simulink model "cassie"  (R2017b)
settings: Solver=FixedStepAuto  StartTime=0.0  StopTime=inf  RelTol=1e-3
InitFcn:
  | PreFunctions.PreParams
undefined symbols (not defined in the file or in its folder): UserParams
libraries: xpcethercatlib x47, ComponentLibrary x10, slrtlib x5, xpcutilitieslib x2, xpcrtudplib x2, dsparch4 x2
(part 1 of 2)
settings Model: xpc_rtwmakecfg_data=_xpcethercatlib_  SimulationMode=external  Creator=hanli  LastModifiedBy=Robot
settings SolverCC: ConcurrentTasks=on  AutoInsertRateTranBlk=on
settings DataIOCC: SaveFormat=StructureWithTime
settings OptimizationCC: BlockReduction=off  SimCompilerOptimization=on  AccelVerboseBuild=on
settings DebuggingCC: InheritedTsInSrcMsg=none
settings HardwareCC: ProdBitPerPointer=32  ProdBitPerSizeT=32  ProdBitPerPtrDiffT=32  ProdLargestAtomicFloat=None  ProdWordSize=32  ProdLongLongMode=on  ProdHWDeviceType=Generic->32-bit x86 compatible
settings RTWCC: SystemTargetFile=slrt.tlc  TemplateMakefile=slrt_default_tmf  Description=Simulink Real-Time  CustomSource=Jp_toe_joint_right_src.c  CodeExecutionProfiling=on  RTWCompilerOptimization=on
settings SimulinkRealTimeCC: SupportVariableSizeSignals=on  RL32LogTETModifier=off  xPCConcurrentTasks=on

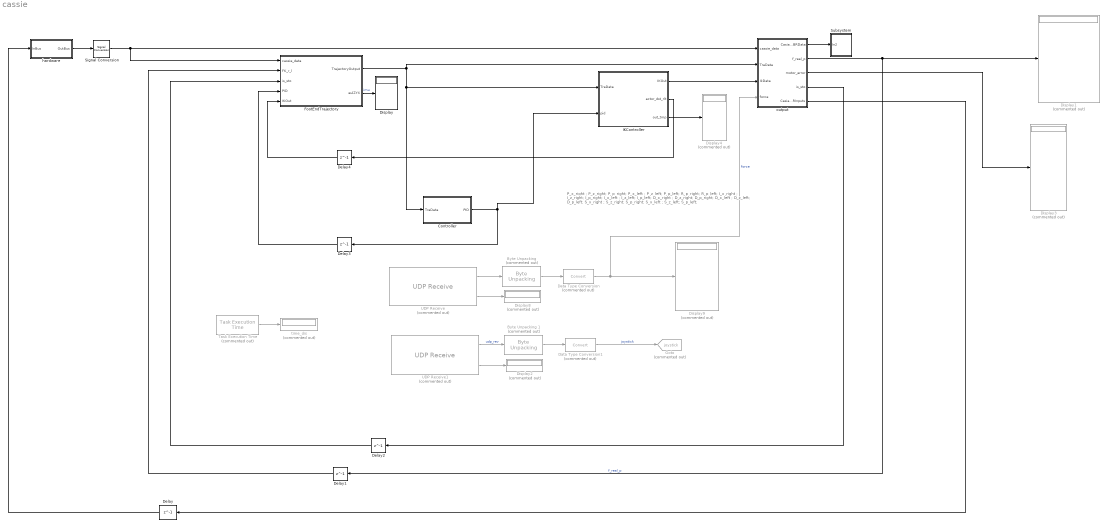
== system cassie ==
  note: P_x_right ; P_z_right; P_p_right; P_x_left ; P_z_left; P_p_left; R_p_right; R_p_left;
      |
      | I_x_right ;   I_z_right;  I_p_right;  I_x_left ; I_z_left;  I_p_left;
      |
      | D_x_right ; D_z_right; D_p_right; D_x_left ; D_z_left; D_p_left;
      |
      | S_x_right ; S_z_right; S_p_right; S_x_left ; S_z_left; S_p_left;
  "Byte Unpacking " : xpcutilitieslib/Byte Unpacking   Commented=on  MaskUnpackedDataTypes={'single'}  MaskUnpackedDataSizes={[6]}  MaskAlignment=1
      settings: SourceProductName=Simulink Real-Time  SourceProductBaseCode=XP
  Byte Unpacking 1 : xpcutilitieslib/Byte Unpacking   Commented=on  MaskUnpackedDataTypes={'int8'}  MaskUnpackedDataSizes={[11]}  MaskAlignment=1
      settings: SourceProductName=Simulink Real-Time  SourceProductBaseCode=XP
  Controller : Subsystem
  Data Type Conversion : DataTypeConversion  Commented=on
  Data Type Conversion1 : DataTypeConversion  Commented=on
  Delay{,1..4} (5 alike) : Delay  DelayLength=1  InitialCondition=0
  Display : Display
  Display{1..4,8..9} (6 alike) : Display  Commented=on
  FootEndTrajectory : Subsystem
  Goto : Goto  Commented=on  GotoTag=joystick  TagVisibility=global
  IKController : Subsystem
  Signal Conversion : SignalConversion  ConversionOutput=Nonvirtual bus  OutDataTypeStr=Bus: CassieOutBus  OverrideOpt=off
  Subsystem : Subsystem
  "Task Execution Time " : slrtlib/Target Management/Execution Parameters/Task Execution Time   Commented=on  ts=1/2000
      settings: SourceProductName=Simulink Real-Time  SourceProductBaseCode=XP
  UDP Receive : xpcrtudplib/UDP Receive  Commented=on  ipAddressVal=Use host-target connection  localPort=10001  rcvWidth=24  rcvFmAny=on  fmAddress=0.0.0.0  maxUDPQueue=8  sampleTime=0.001
      settings: SourceProductName=Simulink Real-Time
  UDP Receive1 : xpcrtudplib/UDP Receive  Commented=on  ipAddressVal=Use host-target connection  localPort=10001  rcvWidth=11  rcvFmAny=on  fmAddress=0.0.0.0  maxUDPQueue=8  sampleTime=0.005
      settings: SourceProductName=Simulink Real-Time
  hardware : Subsystem  InitFcn=PreFunctions.BusInfos
  output : Subsystem
  time_dis : Display  Commented=on
  wires:
  hardware/1(OutBus) -> Signal Conversion/1
  Delay/1 -> hardware/1(InBus)
  Signal Conversion/1 -> FootEndTrajectory/1(cassie_data), output/1(cassie_data)
  output/3(motor_error) -> Display3/1
  "Task Execution Time "/1 -> time_dis/1
  FootEndTrajectory/1(TrajectoryOutput) -> output/2(TraData), Controller/1(TraData), IKController/1(TraData)
  Delay1/1 -> FootEndTrajectory/2(FK_r_l)
  Delay2/1 -> FootEndTrajectory/3(is_sto)
  FootEndTrajectory/2(eulZYX) -> Display/1  "imu"
  Controller/1(PID) -> IKController/2(pid), Delay3/1
  output/2(f_real_p) -> Delay1/1, Display1/1  "f_real_p"
  IKController/1(IKOut) -> output/3(IkData)
  output/1(CasiaBBRData) -> Subsystem/1(In2)
  output/5(CasiaBBRInputs) -> Delay/1
  output/4(is_sto) -> Delay2/1
  UDP Receive/1 -> "Byte Unpacking "/1
  "Byte Unpacking "/1 -> Data Type Conversion/1
  UDP Receive/2 -> Display8/1
  Data Type Conversion/1 -> output/4(force), Display9/1  "force"
  IKController/3(out_tmp) -> Display4/1
  Delay3/1 -> FootEndTrajectory/4(PID)
  UDP Receive1/1 -> Byte Unpacking 1/1  "udp_rev"
  UDP Receive1/2 -> Display2/1
  Byte Unpacking 1/1 -> Data Type Conversion1/1
  Data Type Conversion1/1 -> Goto/1  "joystick"
  Delay4/1 -> FootEndTrajectory/5(IKOut)
  IKController/2(actor_dst_rlt) -> Delay4/1

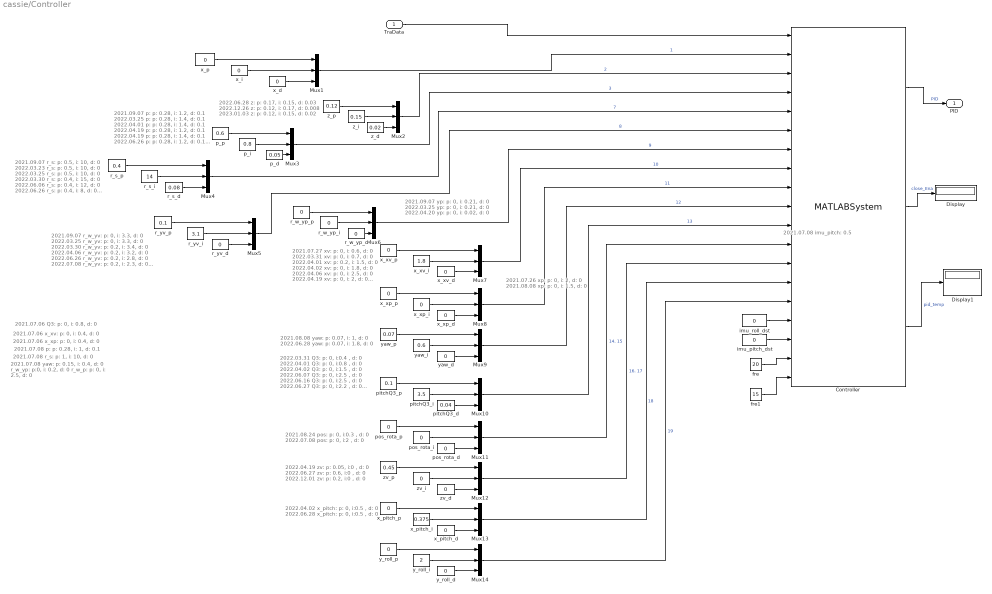
== system cassie/Controller ==
  note: 2021.07.06 x_xp: p: 0, i: 0.4, d: 0
  note: 2021.07.06 x_xv: p: 0, i: 0.4, d: 0
  note: 2021.07.06 Q3: p: 0, i: 0.8, d: 0
  note: 2021.07.08 imu_pitch: 0.5
  note: 2021.07.08 p: p: 0.28, i: 1, d: 0.1
  note: 2021.07.08 r_s: p: 1, i: 10, d: 0
  note: 2021.07.08    yaw: p: 0.15, i: 0.4, d: 0
      |                    r_w_yp: p:0, i: 0.2, d: 0
      |    			r_w_p: p: 0, i: 2.5, d: 0
  note: 2021.07.26     xp: p: 0, i: 2, d: 0
      | 2021.08.08     xp: p: 0, i: 1.5, d: 0
  note: 2021.07.27     xv: p: 0, i: 0.6, d: 0
      | 2022.03.31     xv: p: 0, i: 0.7, d: 0
      | 2022.04.01     xv: p: 0.2, i: 1.5, d: 0
      | 2022.04.02     xv: p: 0, i: 1.8, d: 0
      | 2022.04.06     xv: p: 0, i: 2.5, d: 0
      | 2022.04.19     xv: p: 0, i: 2, d: 0
      | 2022.06.08     xv: p: 0, i: 2, d: 0
      | 2022.06.16     xv: p: 0, i: 2.5, d: 0
      | 2022.06.26     xv: p: 0, i: 2.5, d: 0
      | 2022.07.08     xv: p: 0, i: 1.7, d: 0
  note: 2021.08.08     yaw: p: 0.07, i: 1, d: 0
      | 2022.06.28     yaw: p: 0.07, i: 1.8, d: 0
  note: 2021.09.07     yp: p: 0, i: 0.21, d: 0
      | 2022.03.25     yp: p: 0, i: 0.21, d: 0
      | 2022.04.20     yp: p: 0, i: 0.02, d: 0
  note: 2021.09.07    r_s: p: 0.5, i: 10, d: 0
      | 2022.03.23    r_s: p: 0.5, i: 10, d: 0
      | 2022.03.25    r_s: p: 0.5, i: 10, d: 0
      | 2022.03.30    r_s: p: 0.4, i: 15, d: 0
      | 2022.06.06    r_s: p: 0.4, i: 12, d: 0
      | 2022.06.26    r_s: p: 0.4, i: 8, d: 0
      | 2022.06.28    r_s: p: 0.4, i: 12, d: 0
      | 2022.11.24    r_s: p: 0.4, i: 12, d: 0
      | 2022.12.08    r_s: p: 0.7, i: 16, d: 0.12
      | 2022.12.22    r_s: p: 0.4, i: 16, d: 0.12
      | 2022.12.26    r_s: p: 0.4, i: 14, d: 0.06
  note: 2021.08.24    pos: p: 0, i:0.3 , d: 0
      | 2022.07.08    pos: p: 0, i:2 , d: 0
  note: 2021.09.07     p: p: 0.28, i: 1.2, d: 0.1
      | 2022.03.25     p: p: 0.28, i: 1.4, d: 0.1
      | 2022.04.01     p: p: 0.28, i: 1.4, d: 0.1
      | 2022.04.19     p: p: 0.28, i: 1.2, d: 0.1
      | 2022.04.19     p: p: 0.28, i: 1.4, d: 0.1
      | 2022.06.26     p: p: 0.28, i: 1.2, d: 0.1
      | 2022.06.28     p: p: 0.25, i: 1.4, d: 0.1
  note: 2021.09.07    r_w_yv: p: 0, i: 3.3, d: 0
      | 2022.03.25    r_w_yv: p: 0, i: 3.3, d: 0
      | 2022.03.30    r_w_yv: p: 0.2, i: 3.4, d: 0
      | 2022.04.06    r_w_yv: p: 0.2, i: 3.2, d: 0
      | 2022.06.26    r_w_yv: p: 0.2, i: 2.8, d: 0
      | 2022.07.08    r_w_yv: p: 0.2, i: 2.3, d: 0
      | 2022.08.08    r_w_yv: p: 0.2, i: 2.2, d: 0
      | 2022.12.26    r_w_yv: p: 0, i: 4.2, d: 0
  note: 2022.03.31     Q3: p: 0, i:0.4 , d: 0
      | 2022.04.01     Q3: p: 0, i:0.8 , d: 0
      | 2022.04.02     Q3: p: 0, i:1.5 , d: 0
      | 2022.06.07     Q3: p: 0, i:2.5 , d: 0
      | 2022.06.16     Q3: p: 0, i:2.5 , d: 0
      | 2022.06.27     Q3: p: 0, i:2.2 , d: 0
      | 2022.07.08     Q3: p: 0, i:1.8 , d: 0
      | 2022.12.02     Q3: p: 0, i:2.7 , d: 0
      | 2022.12.07     Q3: p: 0, i:4 , d: 0
      | 2022.12.26     Q3: p: 0.1, i:4 , d: 0.035
  note: 2022.04.02    x_pitch: p: 0, i:0.5 , d: 0
      | 2022.06.28    x_pitch: p: 0, i:0.5 , d: 0
  note: 2022.04.19    zv: p: 0.05, i:0 , d: 0
      | 2022.06.27    zv: p: 0.6, i:0 , d: 0
      | 2022.12.01    zv: p: 0.2, i:0 , d: 0
  note: 2022.06.28     z: p: 0.17, i: 0.15, d: 0.03
      | 2022.12.26     z: p: 0.12, i: 0.17, d: 0.008
      | 2023.01.03     z: p: 0.12, i: 0.15, d: 0.02
  TraData : Inport
  Controller : MATLABSystem  System=Controller  SimulateUsing=Code generation
      mask Type: Controller
      mask Display:
      | disp('Controller');
      | port_label('input',1,'TraData');
      | port_label('input',2,'x_pid');
      | port_label('input',3,'z_pid');
      | port_label('input',4,'p_pid');
      | port_label('input',5,'r_st_pid');
      | port_label('input',6,'yv_pid');
      | port_label('input',7,'yp_pid');
      | port_label('input',8,'xv_pid');
      | port_label('input',9,'xp_pid');
      | port_label('input',10,'yaw_pid');
      | port_label('input',11,'q3_pid');
      | port_label('input',12,'pos_rota_pid');
      | port_label('input',13,'zv_pid');
      | port_label('input',14,'x_pitch_pid');
      | port_label('input',15,'y_roll_pid');
      | port_label('input',16,'imu_roll_dst');
      | port_label('input',17,'imu_pitch_dst');
      | port_label('input',18,'fre_roll');
      | port_label('input',19,'fre_pitch');
      | port_label('output',1,'pid_out');
      | port_label('output',2,'closedloop_Ena');
      | port_label('output',3,'pid_tmp');
  Display : Display
  Display1 : Display
  Mux{1..14} (14 alike) : Mux  Inputs=3
  fre : Constant  Value=20
  fre1 : Constant  Value=15
  imu_pitch_dst : Constant  Value=0
  imu_roll_dst : Constant  Value=0
  p_d : Constant  Value=0.05
  p_i : Constant  Value=0.8
  p_p : Constant  Value=0.6
  pitchQ3_d : Constant  Value=0.04
  pitchQ3_i : Constant  Value=3.5
  pitchQ3_p : Constant  Value=0.1
  pos_rota_d : Constant  Value=0
  pos_rota_i : Constant  Value=0
  pos_rota_p : Constant  Value=0
  r_s_d : Constant  Value=0.08
  r_s_i : Constant  Value=14
  r_s_p : Constant  Value=0.4
  r_w_yp_d : Constant  Value=0
  r_w_yp_i : Constant  Value=0
  r_w_yp_p : Constant  Value=0
  r_yv_d : Constant  Value=0
  r_yv_i : Constant  Value=3.1
  r_yv_p : Constant  Value=0.1
  x_d : Constant  Value=0
  x_i : Constant  Value=0
  x_p : Constant  Value=0
  x_pitch_d : Constant  Value=0
  x_pitch_i : Constant  Value=0.375
  x_pitch_p : Constant  Value=0
  x_xp_d : Constant  Value=0
  x_xp_i : Constant  Value=0
  x_xp_p : Constant  Value=0
  x_xv_d : Constant  Value=0
  x_xv_i : Constant  Value=1.8
  x_xv_p : Constant  Value=0
  y_roll_d : Constant  Value=0
  y_roll_i : Constant  Value=2
  y_roll_p : Constant  Value=0
  yaw_d : Constant  Value=0
  yaw_i : Constant  Value=0.6
  yaw_p : Constant  Value=0.07
  z_d : Constant  Value=0.02
  z_i : Constant  Value=0.15
  z_p : Constant  Value=0.12
  zv_d : Constant  Value=0
  zv_i : Constant  Value=0
  zv_p : Constant  Value=0.45
  PID : Outport
  wires:
  Mux2/1 -> Controller/3  "2"
  p_p/1 -> Mux3/1
  z_p/1 -> Mux2/1
  z_d/1 -> Mux2/3
  z_i/1 -> Mux2/2
  Mux1/1 -> Controller/2  "1"
  p_i/1 -> Mux3/2
  x_p/1 -> Mux1/1
  Controller/1 -> PID/1  "PID"
  x_d/1 -> Mux1/3
  p_d/1 -> Mux3/3
  Mux3/1 -> Controller/4  "3"
  x_i/1 -> Mux1/2
  TraData/1 -> Controller/1
  r_s_d/1 -> Mux4/3
  r_s_i/1 -> Mux4/2
  Mux4/1 -> Controller/5  "7"
  r_s_p/1 -> Mux4/1
  r_yv_p/1 -> Mux5/1
  r_yv_d/1 -> Mux5/3
  r_yv_i/1 -> Mux5/2
  Mux5/1 -> Controller/6  "8"
  Controller/2 -> Display/1  "close_Ena"
  Mux8/1 -> Controller/9  "11"
  x_xv_p/1 -> Mux7/1
  x_xp_i/1 -> Mux8/2
  x_xp_p/1 -> Mux8/1
  x_xp_d/1 -> Mux8/3
  Mux7/1 -> Controller/8  "10"
  r_w_yp_p/1 -> Mux6/1
  r_w_yp_i/1 -> Mux6/2
  Mux6/1 -> Controller/7  "9"
  x_xv_i/1 -> Mux7/2
  r_w_yp_d/1 -> Mux6/3
  x_xv_d/1 -> Mux7/3
  yaw_p/1 -> Mux9/1
  yaw_d/1 -> Mux9/3
  Mux9/1 -> Controller/10  "12"
  yaw_i/1 -> Mux9/2
  Mux10/1 -> Controller/11  "13"
  pitchQ3_d/1 -> Mux10/3
  pitchQ3_i/1 -> Mux10/2
  pitchQ3_p/1 -> Mux10/1
  pos_rota_d/1 -> Mux11/3
  pos_rota_i/1 -> Mux11/2
  pos_rota_p/1 -> Mux11/1
  Mux11/1 -> Controller/12  "14. 15"
  zv_d/1 -> Mux12/3
  Mux12/1 -> Controller/13  "16. 17"
  zv_p/1 -> Mux12/1
  zv_i/1 -> Mux12/2
  x_pitch_p/1 -> Mux13/1
  x_pitch_d/1 -> Mux13/3
  Mux13/1 -> Controller/14  "18"
  x_pitch_i/1 -> Mux13/2
  Controller/3 -> Display1/1  "pid_temp"
  imu_roll_dst/1 -> Controller/16
  imu_pitch_dst/1 -> Controller/17
  fre/1 -> Controller/18
  fre1/1 -> Controller/19
  y_roll_p/1 -> Mux14/1
  Mux14/1 -> Controller/15  "19"
  y_roll_d/1 -> Mux14/3
  y_roll_i/1 -> Mux14/2

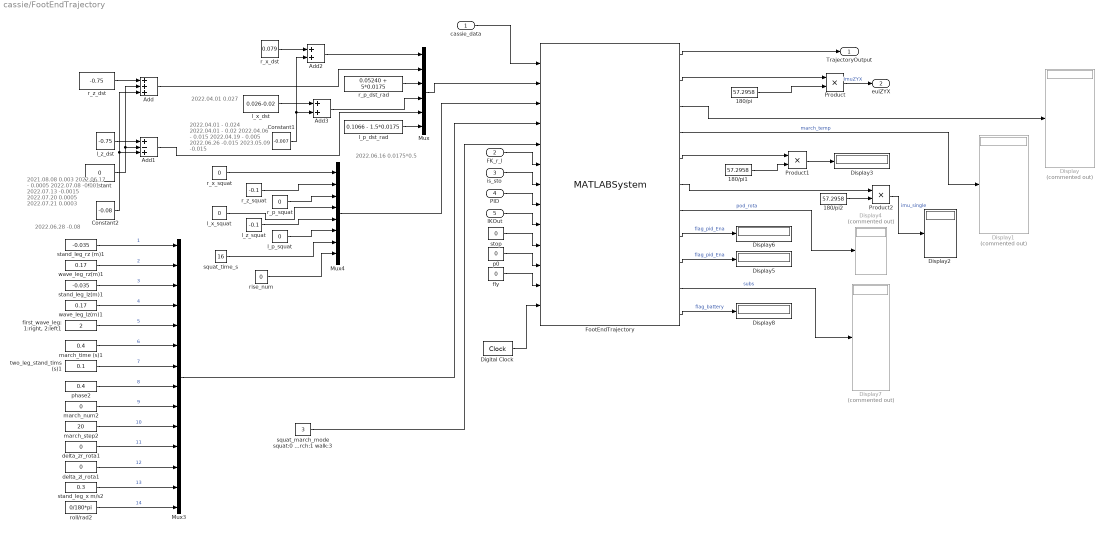
== system cassie/FootEndTrajectory ==
  note: 2021.08.08    0.003
      | 2022.06.17   - 0.0005
      | 2022.07.08   -0.001
      | 2022.07.13   -0.0015
      | 2022.07.20   0.0005
      | 2022.07.21   0.0003
  note: 2022.04.01   - 0.024
      | 2022.04.01   - 0.02
      | 2022.04.06   - 0.015
      | 2022.04.19   - 0.005
      | 2022.06.26    -0.015
      | 2023.05.09    -0.015
  note: 2022.04.01 0.027
  note: 2022.06.16 0.0175*0.5
  note: 2022.06.28 -0.08
  cassie_data : Inport
  FK_r_l : Inport  Port=2
  is_sto : Inport  Port=3
  PID : Inport  Port=4
  IKOut : Inport  Port=5
  180/pi : Constant  Value=57.2958
  180/pi1 : Constant  Value=57.2958
  180/pi2 : Constant  Value=57.2958
  Add : Sum  Inputs=+++
  Add1 : Sum  Inputs=+-+
  Add2 : Sum
  Add3 : Sum
  Constant : Constant  Value=0
  Constant1 : Constant  Value=-0.007
  Constant2 : Constant  Value=-0.08
  Digital Clock : DigitalClock  SampleTime=UserParams.SampleTime
  Display{,1,4,7} (4 alike) : Display  Commented=on
  Display{2..3,5..6,8} (5 alike) : Display
  FootEndTrajectory : MATLABSystem  System=FootEndTrajectory  SimulateUsing=Code generation
      mask Type: FootEndTrajectory
      mask Display:
      | disp('FootEndTrajectory');
      | port_label('input',1,'cassie_data');
      | port_label('input',2,'IK_tgt');
      | port_label('input',3,'squat');
      | port_label('input',4,'march');
      | port_label('input',5,'op_mode');
      | port_label('input',6,'FK_r_l');
      | port_label('input',7,'is_sto');
      | port_label('input',8,'pid_out');
      | port_label('input',9,'actor_dst_rlt');
      | port_label('input',10,'flag_stop');
      | port_label('input',11,'flag_p0');
      | port_label('input',12,'flag_fly');
      | port_label('input',13,'t');
      | port_label('output',1,'TrajectotyOutput');
      | port_label('output',2,'eulZYX');
      | port_label('output',3,'IK_dst');
      | port_label('output',4,'march_temp');
      | port_label('output',5,'yaw0');
      | port_label('output',6,'eulZYX_single');
      | port_label('output',7,'pos_rota');
      | port_label('output',8,'t_pid_Ena');
      | port_label('output',9,'flag_pid_Ena');
      | port_label('output',10,'controller');
      | port_label('output',11,'flag_battery');
  Mux : Mux  Inputs=6
  Mux3 : Mux  Inputs=14
  Mux4 : Mux  Inputs=8
  Product : Product
  Product1 : Product
  Product2 : Product
  delta_zl_rota1 : Constant  Value=0
  delta_zr_rota1 : Constant  Value=0
  "first_wave_leg: 1:right, 2:left1" : Constant  Value=2
  fly : Constant  Value=0
  l_p_dst_rad : Constant  Value=0.1066 - 1.5*0.0175
  l_p_squat : Constant  Value=0
  l_x_dst : Constant  Value=0.026-0.02
  l_x_squat : Constant  Value=0
  l_z_dst : Constant  Value=-0.75
  l_z_squat : Constant  Value=-0.1
  march_num2 : Constant  Value=0
  march_step2 : Constant  Value=20
  march_time (s)1 : Constant  Value=0.4
  p0 : Constant  Value=0
  phase2 : Constant  Value=0.4
  r_p_dst_rad : Constant  Value=0.05240 + 5*0.0175
  r_p_squat : Constant  Value=0
  r_x_dst : Constant  Value=0.079
  r_x_squat : Constant  Value=0
  r_z_dst : Constant  Value=-0.75
  r_z_squat : Constant  Value=-0.1
  rise_num : Constant  Value=0
  roll/rad2 : Constant  Value=0/180*pi
  squat_march_mode squat:0 march:1 walk:3 : Constant  Value=3
  squat_time_s : Constant  Value=16
  stand_leg_lz(m)1 : Constant  Value=-0.035
  stand_leg_rz (m)1 : Constant  Value=-0.035
  stand_leg_x m/s2 : Constant  Value=0.3
  stop : Constant  Value=0
  two_leg_stand_tims (s)1 : Constant  Value=0.1
  wave_leg_lz(m)1 : Constant  Value=0.17
  wave_leg_rz(m)1 : Constant  Value=0.17
  TrajectoryOutput : Outport
  eulZYX : Outport  Port=2
  wires:
  l_z_dst/1 -> Add1/1
  l_x_dst/1 -> Add3/1
  r_x_dst/1 -> Add2/1
  Add1/1 -> Mux/5
  Constant2/1 -> Add1/3, Add/3
  r_x_squat/1 -> Mux4/1
  Constant1/1 -> Add3/2, Add2/2
  r_z_squat/1 -> Mux4/2
  Mux4/1 -> FootEndTrajectory/3
  l_p_squat/1 -> Mux4/6
  is_sto/1 -> FootEndTrajectory/7
  squat_time_s/1 -> Mux4/7
  l_x_squat/1 -> Mux4/4
  r_p_squat/1 -> Mux4/3
  rise_num/1 -> Mux4/8
  FK_r_l/1 -> FootEndTrajectory/6
  FootEndTrajectory/1 -> TrajectoryOutput/1
  l_z_squat/1 -> Mux4/5
  l_p_dst_rad/1 -> Mux/6
  Constant/1 -> Add/2, Add1/2
  Add2/1 -> Mux/1
  r_z_dst/1 -> Add/1
  Add/1 -> Mux/2
  Mux/1 -> FootEndTrajectory/2
  r_p_dst_rad/1 -> Mux/3
  Add3/1 -> Mux/4
  cassie_data/1 -> FootEndTrajectory/1
  Product/1 -> eulZYX/1  "imuZYX"
  FootEndTrajectory/2 -> Product/1
  180/pi/1 -> Product/2
  squat_march_mode squat:0 march:1 walk:3/1 -> FootEndTrajectory/5
  FootEndTrajectory/3 -> Display/1
  PID/1 -> FootEndTrajectory/8
  FootEndTrajectory/4 -> Display1/1  "march_temp"
  IKOut/1 -> FootEndTrajectory/9
  FootEndTrajectory/5 -> Product1/1
  Product1/1 -> Display3/1
  180/pi1/1 -> Product1/2
  FootEndTrajectory/6 -> Product2/1
  180/pi2/1 -> Product2/2
  Product2/1 -> Display2/1  "imu_single"
  FootEndTrajectory/7 -> Display4/1  "pod_rota"
  FootEndTrajectory/9 -> Display5/1  "flag_pid_Ena"
  p0/1 -> FootEndTrajectory/11
  FootEndTrajectory/8 -> Display6/1  "flag_pid_Ena"
  FootEndTrajectory/10 -> Display7/1  "subs"
  FootEndTrajectory/11 -> Display8/1  "flag_battery"
  delta_zr_rota1/1 -> Mux3/11  "11"
  march_time (s)1/1 -> Mux3/6  "6"
  stand_leg_x m/s2/1 -> Mux3/13  "13"
  delta_zl_rota1/1 -> Mux3/12  "12"
  march_step2/1 -> Mux3/10  "10"
  roll/rad2/1 -> Mux3/14  "14"
  phase2/1 -> Mux3/8  "8"
  march_num2/1 -> Mux3/9  "9"
  "first_wave_leg: 1:right, 2:left1"/1 -> Mux3/5  "5"
  stand_leg_lz(m)1/1 -> Mux3/3  "3"
  wave_leg_lz(m)1/1 -> Mux3/4  "4"
  two_leg_stand_tims (s)1/1 -> Mux3/7  "7"
  wave_leg_rz(m)1/1 -> Mux3/2  "2"
  Mux3/1 -> FootEndTrajectory/4
  stand_leg_rz (m)1/1 -> Mux3/1  "1"
  stop/1 -> FootEndTrajectory/10
  fly/1 -> FootEndTrajectory/12
  Digital Clock/1 -> FootEndTrajectory/13

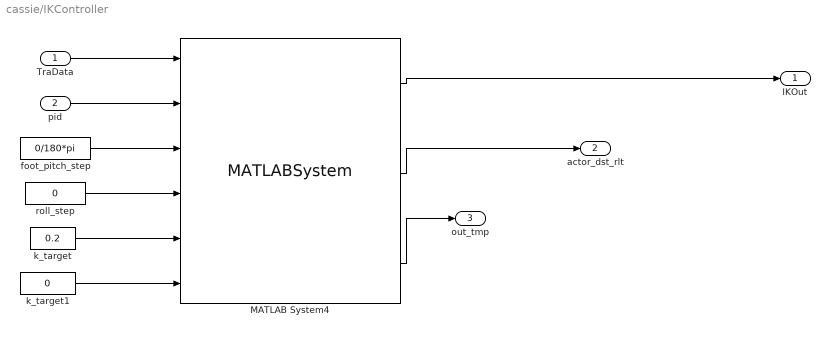
== system cassie/IKController ==
  TraData : Inport
  pid : Inport  Port=2
  MATLAB System4 : MATLABSystem  System=IK_control  right_hip_roll_p=600  right_hip_yaw_p=500  right_hip_pitch_p=600  right_knee_p=600  right_foot_p=200  left_hip_roll_p=600  left_hip_yaw_p=500  left_hip_pitch_p=600  left_knee_p=600  left_foot_p=200  right_hip_roll_d=15  right_hip_yaw_d=2.8  right_hip_pitch_d=6  right_knee_d=12  right_foot_d=3  left_hip_roll_d=15  left_hip_yaw_d=2.8  left_hip_pitch_d=6  left_knee_d=12  left_foot_d=3  Property=[]  Property2=[]  Property3=[]  SimulateUsing=Code generation
      mask Type: IK_control
      mask Display:
      | disp('IK_control');
      | port_label('input',1,'TraData');
      | port_label('input',2,'pid_out');
      | port_label('input',3,'foot_pitch_step');
      | port_label('input',4,'roll_step');
      | port_label('input',5,'k_tgt');
      | port_label('input',6,'q3_dst');
      | port_label('output',1,'IkOut');
      | port_label('output',2,'actor_dst_rlt');
      | port_label('output',3,'out_tmp');
  "foot_pitch_step " : Constant  Value=0/180*pi
  k_target : Constant  Value=0.2
  k_target1 : Constant  Value=0
  roll_step : Constant  Value=0
  IKOut : Outport
  actor_dst_rlt : Outport  Port=2
  out_tmp : Outport  Port=3
  wires:
  TraData/1 -> MATLAB System4/1
  pid/1 -> MATLAB System4/2
  roll_step/1 -> MATLAB System4/4
  MATLAB System4/1 -> IKOut/1
  MATLAB System4/2 -> actor_dst_rlt/1
  MATLAB System4/3 -> out_tmp/1
  k_target/1 -> MATLAB System4/5
  "foot_pitch_step "/1 -> MATLAB System4/3
  k_target1/1 -> MATLAB System4/6

== system cassie/Subsystem ==
  In2 : Inport
  Bus Selector1 : BusSelector  OutputSignals=position,velocity,torque,actTorque,state,tau,f_mode,motor_dst_rlt,imu,fk_r,fk_l,IK_dst,state_march_plan,state_march_real,v_est,p_est,pid,imu_org,s,force,imu_yaw0,s_rl,yaw_est,motor_statusWord,walk_p0,eulZYX_multi,walk_xzdir_wr,walk_xzdir_wl,IK_target,p_pid,motor_statusWord,voltage,temp,ErrorCode,imu_status_word,walk_xv_tgt,walk_xv_dst,con_remote,battery,IK_ry
  "Scope " : slrtlib/Displays and Logging/Scope   scopeno=1  scopetype=File  autostart=on  viewmode=Graphical redraw  formatstr='%15.6f'  grid=on  ylimits=[0,0]  nosamples=2000  noprepostsamples=0  interleave=1  triggermode=FreeRun  triggersignal=1  trigsignalfromport=off  triggerlevel=0.0  triggerslope=Either  triggerscope=1  triggersample=0  filename=H:\CADATA.dat  mode=Commit  writesize=4096  autorestart=on  dynamicfilemode=off  maxwritefilesize=1024*1024^2
  Vector Concatenate1 : Concatenate  NumInputs=40
  wires:
  Bus Selector1/23 -> Vector Concatenate1/23  "<yaw_est>"
  Bus Selector1/12 -> Vector Concatenate1/12  "<IK_dst>"
  Bus Selector1/6 -> Vector Concatenate1/6  "<tau>"
  Bus Selector1/8 -> Vector Concatenate1/8  "<motor_dst_rlt>"
  Bus Selector1/5 -> Vector Concatenate1/5  "<state>"
  Vector Concatenate1/1 -> "Scope "/1
  Bus Selector1/2 -> Vector Concatenate1/2  "<velocity>"
  Bus Selector1/3 -> Vector Concatenate1/3  "<torque>"
  Bus Selector1/9 -> Vector Concatenate1/9  "<imu>"
  Bus Selector1/19 -> Vector Concatenate1/19  "<s>"
  Bus Selector1/18 -> Vector Concatenate1/18  "<imu_org>"
  Bus Selector1/14 -> Vector Concatenate1/14  "<state_march_real>"
  Bus Selector1/20 -> Vector Concatenate1/20  "<force>"
  Bus Selector1/4 -> Vector Concatenate1/4  "<actTorque>"
  Bus Selector1/1 -> Vector Concatenate1/1  "<position>"
  Bus Selector1/25 -> Vector Concatenate1/25  "<walk_p0>"
  Bus Selector1/40 -> Vector Concatenate1/40  "<IK_ry>"
  Bus Selector1/16 -> Vector Concatenate1/16  "<p_est>"
  Bus Selector1/21 -> Vector Concatenate1/21  "<imu_yaw0>"
  Bus Selector1/38 -> Vector Concatenate1/38  "<con_remote>"
  Bus Selector1/39 -> Vector Concatenate1/39  "<battery>"
  In2/1 -> Bus Selector1/1
  Bus Selector1/27 -> Vector Concatenate1/27  "<walk_xzdir_wr>"
  Bus Selector1/24 -> Vector Concatenate1/24  "<motor_statusWord>"
  Bus Selector1/22 -> Vector Concatenate1/22  "<s_rl>"
  Bus Selector1/13 -> Vector Concatenate1/13  "<state_march_plan>"
  Bus Selector1/29 -> Vector Concatenate1/29  "<IK_target>"
  Bus Selector1/36 -> Vector Concatenate1/36  "<walk_xv_tgt>"
  Bus Selector1/31 -> Vector Concatenate1/31  "<motor_statusWord>"
  Bus Selector1/30 -> Vector Concatenate1/30  "<p_pid>"
  Bus Selector1/34 -> Vector Concatenate1/34  "<ErrorCode>"
  Bus Selector1/33 -> Vector Concatenate1/33  "<temp>"
  Bus Selector1/15 -> Vector Concatenate1/15  "<v_est>"
  Bus Selector1/32 -> Vector Concatenate1/32  "<voltage>"
  Bus Selector1/35 -> Vector Concatenate1/35  "<imu_status_word>"
  Bus Selector1/37 -> Vector Concatenate1/37  "<walk_xv_dst>"
  Bus Selector1/10 -> Vector Concatenate1/10  "<fk_r>"
  Bus Selector1/26 -> Vector Concatenate1/26  "<eulZYX_multi>"
  Bus Selector1/28 -> Vector Concatenate1/28  "<walk_xzdir_wl>"
  Bus Selector1/11 -> Vector Concatenate1/11  "<fk_l>"
  Bus Selector1/17 -> Vector Concatenate1/17  "<pid>"
  Bus Selector1/7 -> Vector Concatenate1/7  "<f_mode>"

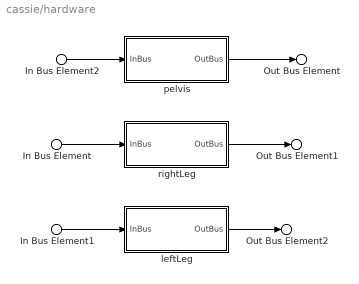
== system cassie/hardware ==
  In Bus Element1 : Inport  PortName=InBus  Element=leftLeg
  In Bus Element : Inport  PortName=InBus  Element=rightLeg
  In Bus Element2 : Inport  PortName=InBus  Element=pelvis
  leftLeg : Subsystem
  pelvis : Subsystem
  rightLeg : Subsystem
  Out Bus Element : Outport  PortName=OutBus  Element=pelvis
  Out Bus Element2 : Outport  PortName=OutBus  Element=leftLeg
  Out Bus Element1 : Outport  PortName=OutBus  Element=rightLeg
  wires:
  pelvis/1(OutBus) -> Out Bus Element/1
  leftLeg/1(OutBus) -> Out Bus Element2/1
  In Bus Element1/1 -> leftLeg/1(InBus)
  rightLeg/1(OutBus) -> Out Bus Element1/1
  In Bus Element/1 -> rightLeg/1(InBus)
  In Bus Element2/1 -> pelvis/1(InBus)

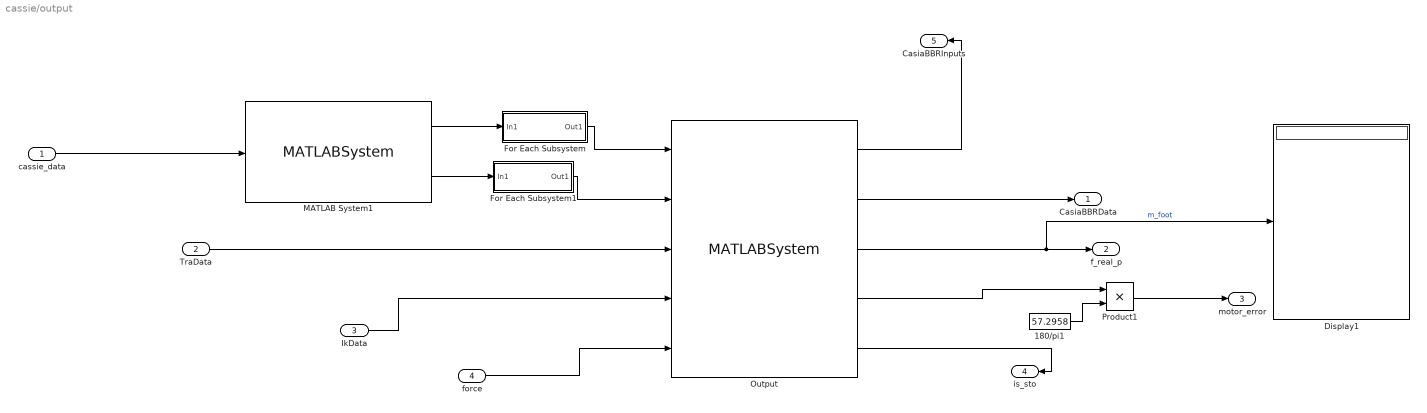
== system cassie/output ==
  cassie_data : Inport
  TraData : Inport  Port=2
  IkData : Inport  Port=3
  force : Inport  Port=4
  180/pi1 : Constant  Value=57.2958
  Display1 : Display
  For Each Subsystem : Subsystem  TreatAsAtomicUnit=on
  For Each Subsystem1 : Subsystem  TreatAsAtomicUnit=on
  MATLAB System1 : MATLABSystem  System=VelocityCurrentFilter  SimulateUsing=Code generation
      mask Type: VelocityCurrentFilter
      mask Display:
      | disp('VelocityCurrentFilter');
      | port_label('input',1,'cassie_data');
      | port_label('output',1,'FilterVelocity');
      | port_label('output',2,'FilrerCurrentPerUnit');
  Output : MATLABSystem  System=Output  SimulateUsing=Code generation
      mask Type: Output
      mask Display:
      | disp('Output');
      | port_label('input',1,'filter_velocity');
      | port_label('input',2,'filter_currentPerUnit');
      | port_label('input',3,'TraData');
      | port_label('input',4,'IkData');
      | port_label('input',5,'force');
      | port_label('output',1,'CasiaBBRInputs');
      | port_label('output',2,'CasiaBBRData');
      | port_label('output',3,'f_real_p');
      | port_label('output',4,'motor_error');
      | port_label('output',5,'is_sto');
  Product1 : Product
  CasiaBBRData : Outport
  f_real_p : Outport  Port=2
  motor_error : Outport  Port=3
  is_sto : Outport  Port=4
  CasiaBBRInputs : Outport  Port=5
  wires:
  IkData/1 -> Output/4
  Product1/1 -> motor_error/1
  Output/5 -> is_sto/1
  MATLAB System1/1 -> For Each Subsystem/1(In1)
  For Each Subsystem/1(Out1) -> Output/1
  MATLAB System1/2 -> For Each Subsystem1/1(In1)
  Output/1 -> CasiaBBRInputs/1
  For Each Subsystem1/1(Out1) -> Output/2
  Output/2 -> CasiaBBRData/1
  Output/3 -> Display1/1, f_real_p/1  "m_foot"
  cassie_data/1 -> MATLAB System1/1
  TraData/1 -> Output/3
  180/pi1/1 -> Product1/2
  Output/4 -> Product1/1
  force/1 -> Output/5

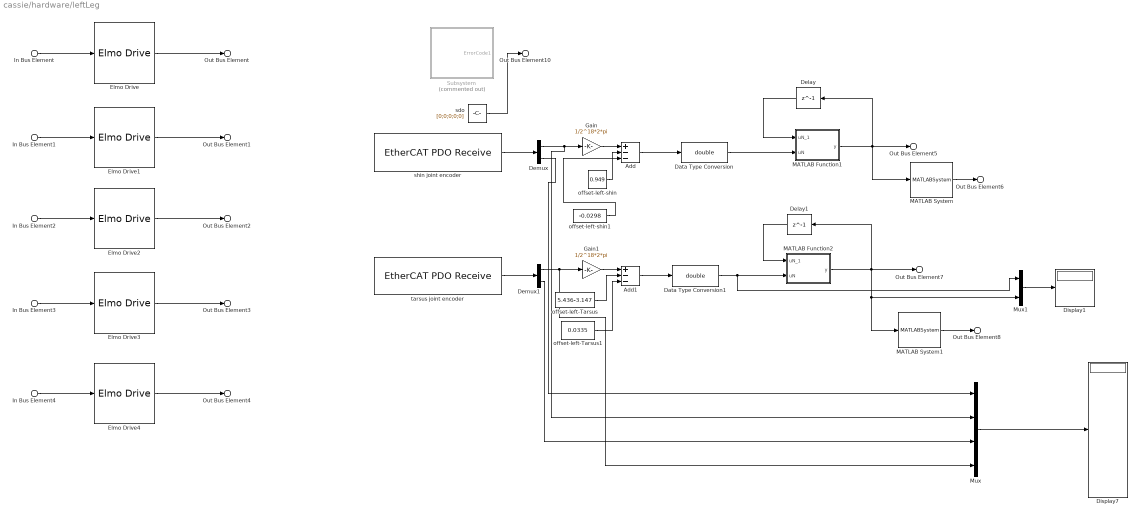
== system cassie/hardware/leftLeg ==
  In Bus Element4 : Inport  PortName=InBus  Element=footDrive
  In Bus Element : Inport  PortName=InBus  Element=hipRollDrive
  In Bus Element1 : Inport  PortName=InBus  Element=hipYawDrive
  In Bus Element2 : Inport  PortName=InBus  Element=hipPitchDrive
  In Bus Element3 : Inport  PortName=InBus  Element=kneeDrive
  Add : Sum  Inputs=+--
  Add1 : Sum  Inputs=+--
  Data Type Conversion : DataTypeConversion  OutDataTypeStr=double
  Data Type Conversion1 : DataTypeConversion  OutDataTypeStr=double
  Delay : Delay  DelayLength=1
  Delay1 : Delay  DelayLength=1
  Demux : Demux  Outputs=2
  Demux1 : Demux  Outputs=2
  Display1 : Display
  Display7 : Display
  Elmo Drive : ComponentLibrary/RealTime/Elmo Drive  ethercatName=LeftHipRoll  slaveAddress=1010  currentLimit=65  gearRatio=1  encoderCounts=2^18  Offset=132170
      link override Mode of Operation PDO Transmit: sig_name=LeftHipRoll.Outputs.Modes of operation  sig_offset=2160  sig_type=int8  sample_time=0.001000
  Elmo Drive1 : ComponentLibrary/RealTime/Elmo Drive  ethercatName=LeftHipYaw  slaveAddress=1011  currentLimit=11.31  gearRatio=1  encoderCounts=2^19  Offset=192617
  Elmo Drive2 : ComponentLibrary/RealTime/Elmo Drive  ethercatName=LeftHipPitch  slaveAddress=1012  currentLimit=65  gearRatio=1  encoderCounts=2^20  Offset=406944
  Elmo Drive3 : ComponentLibrary/RealTime/Elmo Drive  ethercatName=LeftKnee  slaveAddress=1013  currentLimit=65  gearRatio=1  encoderCounts=2^20  Offset=728370
  Elmo Drive4 : ComponentLibrary/RealTime/Elmo Drive  ethercatName=LeftFoot  slaveAddress=1014  currentLimit=7.07  gearRatio=1  encoderCounts=2^19  Offset=282822
  Gain : Gain  Gain=1/2^18*2*pi  ParamDataTypeStr=double  OutDataTypeStr=double
  Gain1 : Gain  Gain=1/2^18*2*pi  ParamDataTypeStr=double  OutDataTypeStr=double
  MATLAB Function1 : MATLAB Function  TreatAsAtomicUnit=on
  MATLAB Function2 : MATLAB Function  TreatAsAtomicUnit=on
  MATLAB System : MATLABSystem  System=FilterSystem  a=[1 -1.76575295625865 0.790448801800725]  b=[12.3479227710395 12.3479227710395 -12.3479227710395 -12.3479227710395]  SimulateUsing=Code generation
      mask Type: FilterSystem
      mask Display: disp('Filter');
  MATLAB System1 : MATLABSystem  System=FilterSystem  a=[1 -1.76575295625865 0.790448801800725]  b=[12.3479227710395 12.3479227710395 -12.3479227710395 -12.3479227710395]  SimulateUsing=Code generation
      mask Type: FilterSystem
      mask Display: disp('Filter');
  Mux : Mux
  Mux1 : Mux  Inputs=2
  Subsystem : Subsystem  Commented=on
  offset-left-Tarsus : Constant  Value=5.436-3.147
  offset-left-Tarsus1 : Constant  Value=0.0335
  offset-left-shin : Constant  Value=0.949
  offset-left-shin1 : Constant  Value=-0.0298
  sdo : Constant  Value=[0;0;0;0;0]  OutDataTypeStr=uint16
  shin joint encoder : xpcethercatlib/EtherCAT PDO Receive  Priority=2  sig_name=Term 6 (EL5042).FB Inputs Channel 1.Position  sig_offset=1672  sig_type=uint32  type_size=32  sig_dim=2  device_id=0  sample_time=0.000500
      settings: SourceProductName=Simulink Real-Time  SourceProductBaseCode=XP
  tarsus joint encoder : xpcethercatlib/EtherCAT PDO Receive  Priority=2  sig_name=Term 6 (EL5042).FB Inputs Channel 2.Position  sig_offset=1752  sig_type=uint32  type_size=32  sig_dim=2  device_id=0  sample_time=0.000500
      settings: SourceProductName=Simulink Real-Time  SourceProductBaseCode=XP
  Out Bus Element : Outport  PortName=OutBus  Element=hipRollDrive
  Out Bus Element1 : Outport  PortName=OutBus  Element=hipYawDrive
  Out Bus Element2 : Outport  PortName=OutBus  Element=hipPitchDrive
  Out Bus Element3 : Outport  PortName=OutBus  Element=kneeDrive
  Out Bus Element4 : Outport  PortName=OutBus  Element=footDrive
  Out Bus Element5 : Outport  PortName=OutBus  Element=shinJoint.position
  Out Bus Element6 : Outport  PortName=OutBus  Element=shinJoint.velocity
  Out Bus Element7 : Outport  PortName=OutBus  Element=tarsusJoint.position
  Out Bus Element8 : Outport  PortName=OutBus  Element=tarsusJoint.velocity
  Out Bus Element10 : Outport  PortName=OutBus  Element=ErrorCode
  wires:
  In Bus Element/1 -> Elmo Drive/1
  Elmo Drive/1 -> Out Bus Element/1
  In Bus Element1/1 -> Elmo Drive1/1
  Elmo Drive1/1 -> Out Bus Element1/1
  In Bus Element2/1 -> Elmo Drive2/1
  Elmo Drive2/1 -> Out Bus Element2/1
  In Bus Element3/1 -> Elmo Drive3/1
  Elmo Drive3/1 -> Out Bus Element3/1
  In Bus Element4/1 -> Elmo Drive4/1
  Elmo Drive4/1 -> Out Bus Element4/1
  MATLAB System/1 -> Out Bus Element6/1
  MATLAB System1/1 -> Out Bus Element8/1
  shin joint encoder/1 -> Demux/1
  Demux/1 -> Mux/2, Gain/1
  tarsus joint encoder/1 -> Demux1/1
  Demux/2 -> Mux/1
  Add1/1 -> Data Type Conversion1/1
  Demux1/1 -> Mux/4, Gain1/1
  offset-left-shin/1 -> Add/2
  Gain/1 -> Add/1
  offset-left-Tarsus/1 -> Add1/2
  Gain1/1 -> Add1/1
  Add/1 -> Data Type Conversion/1
  offset-left-shin1/1 -> Add/3
  offset-left-Tarsus1/1 -> Add1/3
  Data Type Conversion/1 -> MATLAB Function1/2(uN)
  Delay/1 -> MATLAB Function1/1(uN_1)
  MATLAB Function1/1(y) -> Delay/1, Out Bus Element5/1, MATLAB System/1
  sdo/1 -> Out Bus Element10/1
  Mux/1 -> Display7/1
  Demux1/2 -> Mux/3
  Data Type Conversion1/1 -> MATLAB Function2/2(uN), Mux1/1
  Mux1/1 -> Display1/1
  MATLAB Function2/1(y) -> Mux1/2, MATLAB System1/1, Delay1/1, Out Bus Element7/1
  Delay1/1 -> MATLAB Function2/1(uN_1)

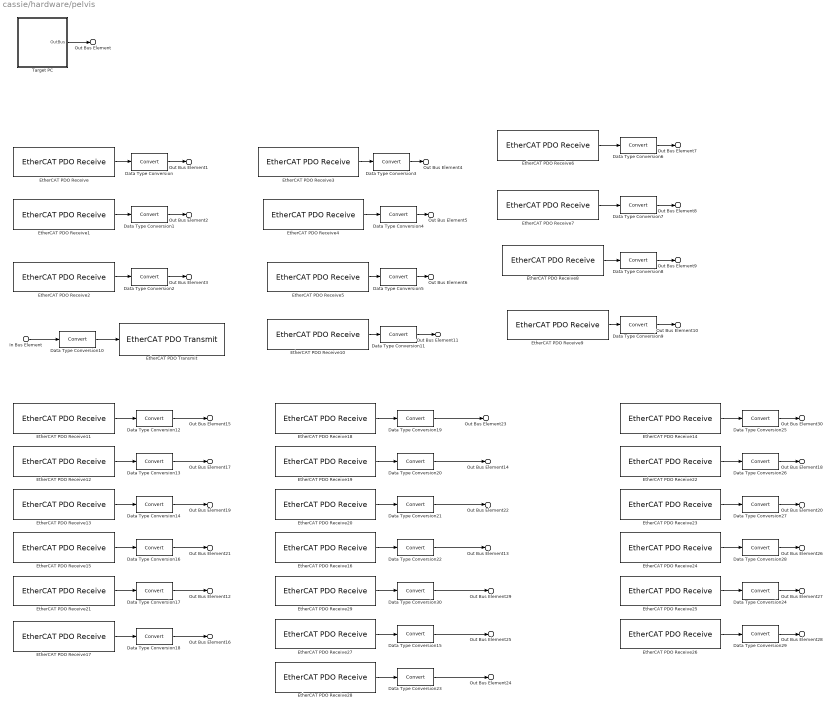
== system cassie/hardware/pelvis ==
  In Bus Element : Inport  PortName=InBus  Element=sto
  Data Type Conversion{,1..30} (31 alike) : DataTypeConversion
  EtherCAT PDO Receive : xpcethercatlib/EtherCAT PDO Receive  Priority=2  sig_name=Box 3 (imu_ethercat_2).Inputs.acc_x  sig_offset=1048  sig_type=single  type_size=32  sig_dim=1  device_id=0  sample_time=0.000500
      settings: SourceProductName=Simulink Real-Time  SourceProductBaseCode=XP
  EtherCAT PDO Receive1 : xpcethercatlib/EtherCAT PDO Receive  Priority=2  sig_name=Box 3 (imu_ethercat_2).Inputs.acc_y  sig_offset=1080  sig_type=single  type_size=32  sig_dim=1  device_id=0  sample_time=0.000500
      settings: SourceProductName=Simulink Real-Time  SourceProductBaseCode=XP
  EtherCAT PDO Receive10 : xpcethercatlib/EtherCAT PDO Receive  Priority=2  sig_name=Box 3 (imu_ethercat_2).Inputs.status_word  sig_offset=1368  sig_type=uint32  type_size=32  sig_dim=1  device_id=0  sample_time=0.000500
      settings: SourceProductName=Simulink Real-Time  SourceProductBaseCode=XP
  EtherCAT PDO Receive11 : xpcethercatlib/EtherCAT PDO Receive  Priority=2  sig_name=Box 1 (sbus).Inputs.ch_0  sig_offset=568  sig_type=uint16  type_size=16  sig_dim=1  device_id=0  sample_time=0.000500
      settings: SourceProductName=Simulink Real-Time  SourceProductBaseCode=XP
  EtherCAT PDO Receive12 : xpcethercatlib/EtherCAT PDO Receive  Priority=2  sig_name=Box 1 (sbus).Inputs.ch_1  sig_offset=584  sig_type=uint16  type_size=16  sig_dim=1  device_id=0  sample_time=0.000500
      settings: SourceProductName=Simulink Real-Time  SourceProductBaseCode=XP
  EtherCAT PDO Receive13 : xpcethercatlib/EtherCAT PDO Receive  Priority=2  sig_name=Box 1 (sbus).Inputs.ch_3  sig_offset=616  sig_type=uint16  type_size=16  sig_dim=1  device_id=0  sample_time=0.000500
      settings: SourceProductName=Simulink Real-Time  SourceProductBaseCode=XP
  EtherCAT PDO Receive14 : xpcethercatlib/EtherCAT PDO Receive  Priority=2  sig_name=Box 2 (battery_info).Inputs.battery_capacity  sig_offset=984  sig_type=single  type_size=32  sig_dim=1  device_id=0  sample_time=0.000500
      settings: SourceProductName=Simulink Real-Time  SourceProductBaseCode=XP
  EtherCAT PDO Receive15 : xpcethercatlib/EtherCAT PDO Receive  Priority=2  sig_name=Box 1 (sbus).Inputs.ch_4  sig_offset=632  sig_type=uint16  type_size=16  sig_dim=1  device_id=0  sample_time=0.000500
      settings: SourceProductName=Simulink Real-Time  SourceProductBaseCode=XP
  EtherCAT PDO Receive16 : xpcethercatlib/EtherCAT PDO Receive  Priority=2  sig_name=Box 1 (sbus).Inputs.ch_5  sig_offset=648  sig_type=uint16  type_size=16  sig_dim=1  device_id=0  sample_time=0.000500
      settings: SourceProductName=Simulink Real-Time  SourceProductBaseCode=XP
  EtherCAT PDO Receive17 : xpcethercatlib/EtherCAT PDO Receive  Priority=2  sig_name=Box 1 (sbus).Inputs.ch_6  sig_offset=664  sig_type=uint16  type_size=16  sig_dim=1  device_id=0  sample_time=0.000500
      settings: SourceProductName=Simulink Real-Time  SourceProductBaseCode=XP
  EtherCAT PDO Receive18 : xpcethercatlib/EtherCAT PDO Receive  Priority=2  sig_name=Box 1 (sbus).Inputs.ch_7  sig_offset=680  sig_type=uint16  type_size=16  sig_dim=1  device_id=0  sample_time=0.000500
      settings: SourceProductName=Simulink Real-Time  SourceProductBaseCode=XP
  EtherCAT PDO Receive19 : xpcethercatlib/EtherCAT PDO Receive  Priority=2  sig_name=Box 1 (sbus).Inputs.ch_8  sig_offset=696  sig_type=uint16  type_size=16  sig_dim=1  device_id=0  sample_time=0.000500
      settings: SourceProductName=Simulink Real-Time  SourceProductBaseCode=XP
  EtherCAT PDO Receive2 : xpcethercatlib/EtherCAT PDO Receive  Priority=2  sig_name=Box 3 (imu_ethercat_2).Inputs.acc_z  sig_offset=1112  sig_type=single  type_size=32  sig_dim=1  device_id=0  sample_time=0.000500
      settings: SourceProductName=Simulink Real-Time  SourceProductBaseCode=XP
  EtherCAT PDO Receive20 : xpcethercatlib/EtherCAT PDO Receive  Priority=2  sig_name=Box 1 (sbus).Inputs.ch_9  sig_offset=712  sig_type=uint16  type_size=16  sig_dim=1  device_id=0  sample_time=0.000500
      settings: SourceProductName=Simulink Real-Time  SourceProductBaseCode=XP
  EtherCAT PDO Receive21 : xpcethercatlib/EtherCAT PDO Receive  Priority=2  sig_name=Box 1 (sbus).Inputs.ch_10  sig_offset=728  sig_type=uint16  type_size=16  sig_dim=1  device_id=0  sample_time=0.000500
      settings: SourceProductName=Simulink Real-Time  SourceProductBaseCode=XP
  EtherCAT PDO Receive22 : xpcethercatlib/EtherCAT PDO Receive  Priority=2  sig_name=Box 2 (battery_info).Inputs.current  sig_offset=920  sig_type=single  type_size=32  sig_dim=1  device_id=0  sample_time=0.000500
      settings: SourceProductName=Simulink Real-Time  SourceProductBaseCode=XP
  EtherCAT PDO Receive23 : xpcethercatlib/EtherCAT PDO Receive  Priority=2  sig_name=Box 2 (battery_info).Inputs.current_capacity  sig_offset=952  sig_type=single  type_size=32  sig_dim=1  device_id=0  sample_time=0.000500
      settings: SourceProductName=Simulink Real-Time  SourceProductBaseCode=XP
  EtherCAT PDO Receive24 : xpcethercatlib/EtherCAT PDO Receive  Priority=2  sig_name=Box 2 (battery_info).Inputs.empty_  sig_offset=1032  sig_type=uint16  type_size=16  sig_dim=1  device_id=0  sample_time=0.000500
      settings: SourceProductName=Simulink Real-Time  SourceProductBaseCode=XP
  EtherCAT PDO Receive25 : xpcethercatlib/EtherCAT PDO Receive  Priority=2  sig_name=Box 2 (battery_info).Inputs.protect_status  sig_offset=1016  sig_type=uint16  type_size=16  sig_dim=1  device_id=0  sample_time=0.000500
      settings: SourceProductName=Simulink Real-Time  SourceProductBaseCode=XP
  EtherCAT PDO Receive26 : xpcethercatlib/EtherCAT PDO Receive  Priority=2  sig_name=Box 2 (battery_info).Inputs.voltage  sig_offset=888  sig_type=single  type_size=32  sig_dim=1  device_id=0  sample_time=0.000500
      settings: SourceProductName=Simulink Real-Time  SourceProductBaseCode=XP
  EtherCAT PDO Receive27 : xpcethercatlib/EtherCAT PDO Receive  Priority=2  sig_name=Box 1 (sbus).Inputs.fail_safe  sig_offset=872  sig_type=uint16  type_size=16  sig_dim=1  device_id=0  sample_time=0.000500
      settings: SourceProductName=Simulink Real-Time  SourceProductBaseCode=XP
  EtherCAT PDO Receive28 : xpcethercatlib/EtherCAT PDO Receive  Priority=2  sig_name=Box 1 (sbus).Inputs.frame_lost  sig_offset=856  sig_type=uint16  type_size=16  sig_dim=1  device_id=0  sample_time=0.000500
      settings: SourceProductName=Simulink Real-Time  SourceProductBaseCode=XP
  EtherCAT PDO Receive29 : xpcethercatlib/EtherCAT PDO Receive  Priority=2  sig_name=Box 1 (sbus).Inputs.ch_12  sig_offset=760  sig_type=uint16  type_size=16  sig_dim=1  device_id=0  sample_time=0.000500
      settings: SourceProductName=Simulink Real-Time  SourceProductBaseCode=XP
  EtherCAT PDO Receive3 : xpcethercatlib/EtherCAT PDO Receive  Priority=2  sig_name=Box 3 (imu_ethercat_2).Inputs.gyr_x  sig_offset=1144  sig_type=single  type_size=32  sig_dim=1  device_id=0  sample_time=0.000500
      settings: SourceProductName=Simulink Real-Time  SourceProductBaseCode=XP
  EtherCAT PDO Receive4 : xpcethercatlib/EtherCAT PDO Receive  Priority=2  sig_name=Box 3 (imu_ethercat_2).Inputs.gyr_y  sig_offset=1176  sig_type=single  type_size=32  sig_dim=1  device_id=0  sample_time=0.000500
      settings: SourceProductName=Simulink Real-Time  SourceProductBaseCode=XP
  EtherCAT PDO Receive5 : xpcethercatlib/EtherCAT PDO Receive  Priority=2  sig_name=Box 3 (imu_ethercat_2).Inputs.gyr_z  sig_offset=1208  sig_type=single  type_size=32  sig_dim=1  device_id=0  sample_time=0.000500
      settings: SourceProductName=Simulink Real-Time  SourceProductBaseCode=XP
  EtherCAT PDO Receive6 : xpcethercatlib/EtherCAT PDO Receive  Priority=2  sig_name=Box 3 (imu_ethercat_2).Inputs.q0  sig_offset=1240  sig_type=single  type_size=32  sig_dim=1  device_id=0  sample_time=0.000500
      settings: SourceProductName=Simulink Real-Time  SourceProductBaseCode=XP
  EtherCAT PDO Receive7 : xpcethercatlib/EtherCAT PDO Receive  Priority=2  sig_name=Box 3 (imu_ethercat_2).Inputs.q1  sig_offset=1272  sig_type=single  type_size=32  sig_dim=1  device_id=0  sample_time=0.000500
      settings: SourceProductName=Simulink Real-Time  SourceProductBaseCode=XP
  EtherCAT PDO Receive8 : xpcethercatlib/EtherCAT PDO Receive  Priority=2  sig_name=Box 3 (imu_ethercat_2).Inputs.q2  sig_offset=1304  sig_type=single  type_size=32  sig_dim=1  device_id=0  sample_time=0.000500
      settings: SourceProductName=Simulink Real-Time  SourceProductBaseCode=XP
  EtherCAT PDO Receive9 : xpcethercatlib/EtherCAT PDO Receive  Priority=2  sig_name=Box 3 (imu_ethercat_2).Inputs.q3  sig_offset=1336  sig_type=single  type_size=32  sig_dim=1  device_id=0  sample_time=0.000500
      settings: SourceProductName=Simulink Real-Time  SourceProductBaseCode=XP
  "EtherCAT PDO Transmit " : xpcethercatlib/EtherCAT PDO Transmit   Priority=3  sig_name=Box 3 (imu_ethercat_2).Outputs.sto  sig_offset=1048  sig_type=uint8  type_size=8  sig_dim=1  device_id=0  sample_time=0.000500
      settings: SourceProductName=Simulink Real-Time  SourceProductBaseCode=XP
  Target PC : Subsystem  AncestorBlock=ComponentLibrary/RealTime/Target PC  mask{pci_bus=1, pci_slot=0, pci_function=0}
      mask prompts: pci_bus "PCI bus:"; pci_slot "PCI slot:"; pci_function "PCI function:"
      mask TypeOptions pci_bus: EtherCAT Init/pci_bus
      mask TypeOptions pci_slot: EtherCAT Init/pci_slot
      mask TypeOptions pci_function: EtherCAT Init/pci_function
  Out Bus Element : Outport  PortName=OutBus  Element=targetPc
  Out Bus Element1 : Outport  PortName=OutBus  Element=imu.acc_x
  Out Bus Element2 : Outport  PortName=OutBus  Element=imu.acc_y
  Out Bus Element3 : Outport  PortName=OutBus  Element=imu.acc_z
  Out Bus Element4 : Outport  PortName=OutBus  Element=imu.gyr_x
  Out Bus Element5 : Outport  PortName=OutBus  Element=imu.gyr_y
  Out Bus Element6 : Outport  PortName=OutBus  Element=imu.gyr_z
  Out Bus Element7 : Outport  PortName=OutBus  Element=imu.q0
  Out Bus Element8 : Outport  PortName=OutBus  Element=imu.q1
  Out Bus Element9 : Outport  PortName=OutBus  Element=imu.q2
  Out Bus Element10 : Outport  PortName=OutBus  Element=imu.q3
  Out Bus Element11 : Outport  PortName=OutBus  Element=imu.status_word
  Out Bus Element15 : Outport  PortName=OutBus  Element=remote.forward
  Out Bus Element17 : Outport  PortName=OutBus  Element=remote.turn
  Out Bus Element19 : Outport  PortName=OutBus  Element=remote.move
  Out Bus Element21 : Outport  PortName=OutBus  Element=remote.ES
  Out Bus Element12 : Outport  PortName=OutBus  Element=remote.pid
  Out Bus Element16 : Outport  PortName=OutBus  Element=remote.switch24
  Out Bus Element23 : Outport  PortName=OutBus  Element=remote.switch48
  Out Bus Element14 : Outport  PortName=OutBus  Element=remote.op
  Out Bus Element22 : Outport  PortName=OutBus  Element=remote.reset_position
  Out Bus Element13 : Outport  PortName=OutBus  Element=remote.march
  Out Bus Element25 : Outport  PortName=OutBus  Element=remote.fail_safe
  Out Bus Element24 : Outport  PortName=OutBus  Element=remote.frame_lost
  Out Bus Element29 : Outport  PortName=OutBus  Element=remote.rise
  Out Bus Element30 : Outport  PortName=OutBus  Element=battery.battery_capacity
  Out Bus Element18 : Outport  PortName=OutBus  Element=battery.current
  Out Bus Element20 : Outport  PortName=OutBus  Element=battery.current_capacity
  Out Bus Element26 : Outport  PortName=OutBus  Element=battery.empty_
  Out Bus Element27 : Outport  PortName=OutBus  Element=battery.protect_status
  Out Bus Element28 : Outport  PortName=OutBus  Element=battery.voltage
  wires:
  Target PC/1(OutBus) -> Out Bus Element/1
  EtherCAT PDO Receive/1 -> Data Type Conversion/1
  EtherCAT PDO Receive5/1 -> Data Type Conversion5/1
  EtherCAT PDO Receive1/1 -> Data Type Conversion1/1
  EtherCAT PDO Receive2/1 -> Data Type Conversion2/1
  EtherCAT PDO Receive4/1 -> Data Type Conversion4/1
  EtherCAT PDO Receive6/1 -> Data Type Conversion6/1
  EtherCAT PDO Receive7/1 -> Data Type Conversion7/1
  EtherCAT PDO Receive8/1 -> Data Type Conversion8/1
  EtherCAT PDO Receive9/1 -> Data Type Conversion9/1
  EtherCAT PDO Receive3/1 -> Data Type Conversion3/1
  Data Type Conversion/1 -> Out Bus Element1/1
  Data Type Conversion1/1 -> Out Bus Element2/1
  Data Type Conversion2/1 -> Out Bus Element3/1
  Data Type Conversion3/1 -> Out Bus Element4/1
  Data Type Conversion4/1 -> Out Bus Element5/1
  Data Type Conversion5/1 -> Out Bus Element6/1
  Data Type Conversion6/1 -> Out Bus Element7/1
  Data Type Conversion7/1 -> Out Bus Element8/1
  Data Type Conversion8/1 -> Out Bus Element9/1
  Data Type Conversion9/1 -> Out Bus Element10/1
  Data Type Conversion10/1 -> "EtherCAT PDO Transmit "/1
  In Bus Element/1 -> Data Type Conversion10/1
  EtherCAT PDO Receive10/1 -> Data Type Conversion11/1
  Data Type Conversion11/1 -> Out Bus Element11/1
  EtherCAT PDO Receive11/1 -> Data Type Conversion12/1
  EtherCAT PDO Receive12/1 -> Data Type Conversion13/1
  EtherCAT PDO Receive13/1 -> Data Type Conversion14/1
  EtherCAT PDO Receive15/1 -> Data Type Conversion16/1
  EtherCAT PDO Receive17/1 -> Data Type Conversion18/1
  EtherCAT PDO Receive18/1 -> Data Type Conversion19/1
  EtherCAT PDO Receive19/1 -> Data Type Conversion20/1
  EtherCAT PDO Receive20/1 -> Data Type Conversion21/1
  Data Type Conversion12/1 -> Out Bus Element15/1
  Data Type Conversion13/1 -> Out Bus Element17/1
  Data Type Conversion14/1 -> Out Bus Element19/1
  Data Type Conversion16/1 -> Out Bus Element21/1
  Data Type Conversion17/1 -> Out Bus Element12/1
  Data Type Conversion18/1 -> Out Bus Element16/1
  Data Type Conversion19/1 -> Out Bus Element23/1
  Data Type Conversion20/1 -> Out Bus Element14/1
  Data Type Conversion21/1 -> Out Bus Element22/1
  Data Type Conversion22/1 -> Out Bus Element13/1
  Data Type Conversion23/1 -> Out Bus Element24/1
  Data Type Conversion15/1 -> Out Bus Element25/1
  EtherCAT PDO Receive26/1 -> Data Type Conversion29/1
  EtherCAT PDO Receive25/1 -> Data Type Conversion24/1
  Data Type Conversion24/1 -> Out Bus Element27/1
  Data Type Conversion25/1 -> Out Bus Element30/1
  EtherCAT PDO Receive24/1 -> Data Type Conversion28/1
  EtherCAT PDO Receive14/1 -> Data Type Conversion25/1
  EtherCAT PDO Receive22/1 -> Data Type Conversion26/1
  EtherCAT PDO Receive23/1 -> Data Type Conversion27/1
  Data Type Conversion28/1 -> Out Bus Element26/1
  Data Type Conversion27/1 -> Out Bus Element20/1
  Data Type Conversion29/1 -> Out Bus Element28/1
  Data Type Conversion26/1 -> Out Bus Element18/1
  EtherCAT PDO Receive28/1 -> Data Type Conversion23/1
  EtherCAT PDO Receive27/1 -> Data Type Conversion15/1
  EtherCAT PDO Receive21/1 -> Data Type Conversion17/1
  EtherCAT PDO Receive16/1 -> Data Type Conversion22/1
  EtherCAT PDO Receive29/1 -> Data Type Conversion30/1
  Data Type Conversion30/1 -> Out Bus Element29/1
